simulink model "Nozzle_TestBed_org"  (Simulink 10.0)
settings: Solver=FixedStepDiscrete  StartTime=0.0  StopTime=1  FixedStep=1  RelTol=1e-3  EnableMultiTasking=on
undefined symbols (not defined in the file): MWS
libraries: Lib_Turbo_Nozzle_TMATS x1
settings Model: Creator=jwchapm2  LastModifiedBy=annonymous
settings DataIOCC: LimitDataPoints=on
settings OptimizationCC: ExpressionDepthLimit=2147483647
settings DebuggingCC: SolverPrmCheckMsg=warning  StateNameClashWarn=warning
settings GRTTargetCC: GeneratePreprocessorConditionals=Disable all  CombineOutputUpdateFcns=on  GRTInterface=off
settings ConfigComp: CovExternalEMLEnable=off

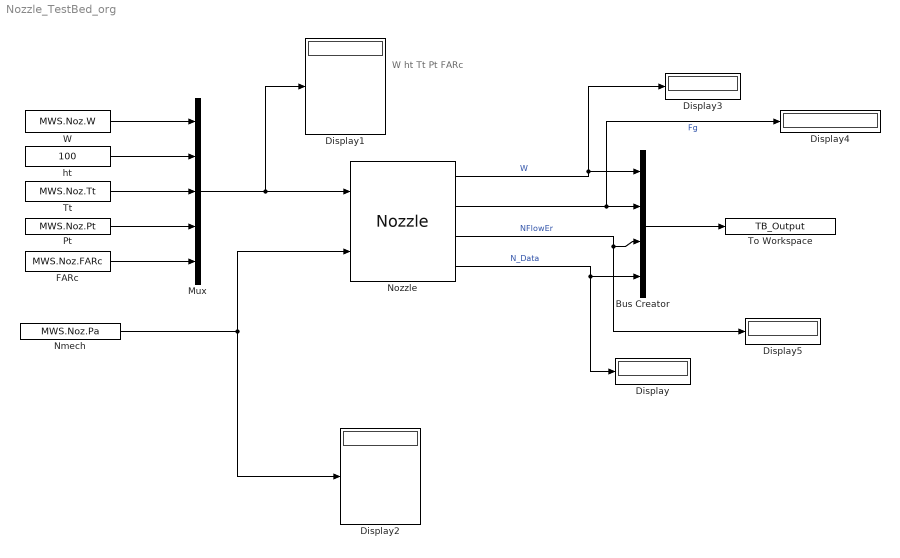
== system Nozzle_TestBed_org ==
  note: W
      | ht
      | Tt
      | Pt
      | FARc
  Bus Creator : BusCreator  Inputs=4
  Display{,1..5} (6 alike) : Display
  FARc : Constant  Value=MWS.Noz.FARc
  Mux : Mux  Inputs=5
  Nmech : Constant  Value=MWS.Noz.Pa
  Nozzle : Lib_Turbo_Nozzle_TMATS/Nozzle  N_TArea_M=MWS.Noz.ATh  N_FL_M=MWS.Noz.LossPerc  X_N_TtVec2_M=MWS.Noz.TtVec  T_N_TGArray_M=MWS.Noz.TGArray  X_N_PEQPaVec_M=MWS.Noz.PeQPaVec  T_N_CdThArray_M=MWS.Noz.CdThArray  X_N_FARVec_M=MWS.Noz.FARVec  T_N_RtArray_M=MWS.Noz.RArray  Y_N_TtVec_M=MWS.Noz.TtVec  T_N_MAP_gammaArray_M=MWS.Noz.GArray  T_N_CvArray_M=MWS.Noz.CvArray  iDesign_M=off  WDes_M=100
  Pt : Constant  Value=MWS.Noz.Pt
  To Workspace : ToWorkspace  VariableName=TB_Output  SampleTime=-1
  Tt : Constant  Value=MWS.Noz.Tt
  W : Constant  Value=MWS.Noz.W
  ht : Constant  Value=100
  wires:
  Nmech/1 -> Display2/1, Nozzle/2
  W/1 -> Mux/1
  FARc/1 -> Mux/5
  Tt/1 -> Mux/3
  Pt/1 -> Mux/4
  Mux/1 -> Display1/1, Nozzle/1
  Nozzle/1 -> Bus Creator/1, Display3/1  "W"
  Nozzle/2 -> Bus Creator/2, Display4/1  "Fg"
  Nozzle/3 -> Bus Creator/3, Display5/1  "NFlowEr"
  Nozzle/4 -> Display/1, Bus Creator/4  "N_Data"
  Bus Creator/1 -> To Workspace/1
  ht/1 -> Mux/2
